simulink model "baselineisp_arch_v1"  (R2023b)
settings: Solver=VariableStepAuto  StartTime=0.0  StopTime=10.0  RelTol=1e-3
model workspace (MAT data in the model file):
  Input = Simulink.Bus
  Input.Alignment = -1
  Input.PreserveElementDimensions = 0
  Input.Elements_internal = Simulink.BusElement
  Input.Elements_internal.DimensionsMode = 'Fixed'
  Input.Elements_internal.SamplingMode = 'Sample based'
  Input.Elements_internal.SampleTime = -1
  Input.Elements_internal.Name = 'RAW'
  Input.Elements_internal.DataType_internal = 'ValueType: RAW'
  Input.Elements_internal.Complexity = 'real'
  Input.Elements_internal.Dimensions = 1
  Input.DataScope = 'Auto'
  RAW = Simulink.ValueType
  RAW.DataType = 'uint16'
settings Model: Creator=csl  LastModifiedBy=csl

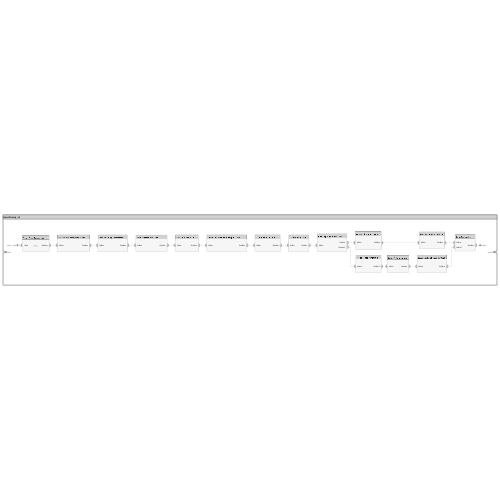
[thumbnail: Simulink's stored preview of the top-level diagram]
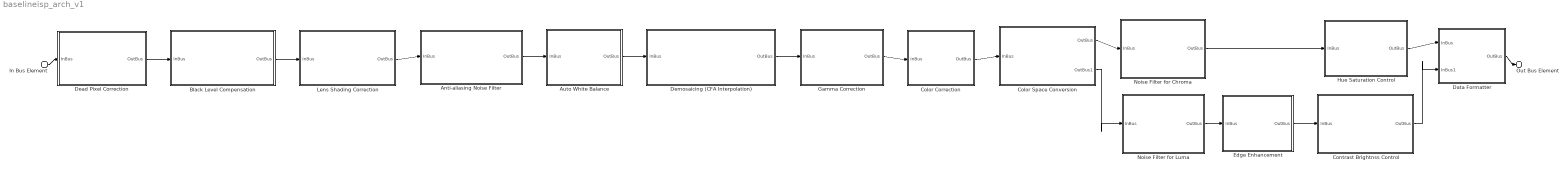
== system baselineisp_arch_v1 ==
  In Bus Element : Inport  PortName=InBus  Element=RAW
  Anti-aliasing Noise Filter : Subsystem
      settings: PortSchema="{\"entries\":[{\"content\":{\"headerSize\":26,\"margin\":15,\"minimumSpacing\":25,\"sides\":[{\"content\":{\"connectorIds\":[\"In1\"]},\"type\":\"ConnectorPlacement.EquallySpacedRectSide\",\"uuid\":\"2ef9bd17-36b9-46a7-9186-123a5b4f1bb0\"},{\"content\":{\"connectorIds\":[\"Out1\"],\"side\":\"RIGHT\"},\"type\":\"ConnectorPlacement.EquallySpacedRectSide\",\"uuid\":\"d5e57a0a-cb8d-4d21-83db-117ffcc7e54f\"},{\"content\":{\"side\":\"TOP\"},\"type\":\"ConnectorPlacement.EquallySpacedRectSide\",\"uuid\":\"a9269390-9b6c-4e98-a738-6052543cf38e\"}]},\"type\":\"ConnectorPlacement.EquallySpacedConnector\",\"uuid\":\"34a5eba8-ed92-482b-8745-835516add4be\"}],\"packageUris\":[\"http://schema.mathworks.com/mf0/Connector/R2020b\"],\"version\":\"1.0\"}"
  Auto White Balance : Subsystem
      settings: PortSchema="{\"entries\":[{\"content\":{\"headerSize\":26,\"margin\":15,\"minimumSpacing\":25,\"sides\":[{\"content\":{\"connectorIds\":[\"In1\"]},\"type\":\"ConnectorPlacement.EquallySpacedRectSide\",\"uuid\":\"2ef9bd17-36b9-46a7-9186-123a5b4f1bb0\"},{\"content\":{\"connectorIds\":[\"Out1\"],\"side\":\"RIGHT\"},\"type\":\"ConnectorPlacement.EquallySpacedRectSide\",\"uuid\":\"d5e57a0a-cb8d-4d21-83db-117ffcc7e54f\"},{\"content\":{\"side\":\"TOP\"},\"type\":\"ConnectorPlacement.EquallySpacedRectSide\",\"uuid\":\"a9269390-9b6c-4e98-a738-6052543cf38e\"},{\"content\":{\"side\":\"BOTTOM\"},\"type\":\"ConnectorPlacement.EquallySpacedRectSide\",\"uuid\":\"7c626892-77ff-47ce-8fd5-626703806efa\"}]},\"type\":\"ConnectorPlacement.EquallySpacedConnector\",\"uuid\":\"34a5eba8-ed92-482b-8745-835516add4be\"}],\"packageUris\":[\"http://schema.mathworks.com/mf0/Connector/R2020b\"],\"version\":\"1.0\"}"
  Black Level Compensation : Subsystem
      settings: PortSchema="{\"entries\":[{\"content\":{\"headerSize\":26,\"margin\":15,\"minimumSpacing\":25,\"sides\":[{\"content\":{\"connectorIds\":[\"In1\"]},\"type\":\"ConnectorPlacement.EquallySpacedRectSide\",\"uuid\":\"2ef9bd17-36b9-46a7-9186-123a5b4f1bb0\"},{\"content\":{\"connectorIds\":[\"Out1\"],\"side\":\"RIGHT\"},\"type\":\"ConnectorPlacement.EquallySpacedRectSide\",\"uuid\":\"d5e57a0a-cb8d-4d21-83db-117ffcc7e54f\"},{\"content\":{\"side\":\"TOP\"},\"type\":\"ConnectorPlacement.EquallySpacedRectSide\",\"uuid\":\"a9269390-9b6c-4e98-a738-6052543cf38e\"}]},\"type\":\"ConnectorPlacement.EquallySpacedConnector\",\"uuid\":\"34a5eba8-ed92-482b-8745-835516add4be\"}],\"packageUris\":[\"http://schema.mathworks.com/mf0/Connector/R2020b\"],\"version\":\"1.0\"}"
  Color Correction : Subsystem
      settings: PortSchema="{\"entries\":[{\"content\":{\"headerSize\":26,\"margin\":15,\"minimumSpacing\":25,\"sides\":[{\"content\":{\"connectorIds\":[\"In1\"]},\"type\":\"ConnectorPlacement.EquallySpacedRectSide\",\"uuid\":\"2ef9bd17-36b9-46a7-9186-123a5b4f1bb0\"},{\"content\":{\"connectorIds\":[\"Out1\"],\"side\":\"RIGHT\"},\"type\":\"ConnectorPlacement.EquallySpacedRectSide\",\"uuid\":\"d5e57a0a-cb8d-4d21-83db-117ffcc7e54f\"},{\"content\":{\"side\":\"TOP\"},\"type\":\"ConnectorPlacement.EquallySpacedRectSide\",\"uuid\":\"a9269390-9b6c-4e98-a738-6052543cf38e\"},{\"content\":{\"side\":\"BOTTOM\"},\"type\":\"ConnectorPlacement.EquallySpacedRectSide\",\"uuid\":\"3fcc8b46-bf35-454b-b542-ea93b895bca3\"}]},\"type\":\"ConnectorPlacement.EquallySpacedConnector\",\"uuid\":\"34a5eba8-ed92-482b-8745-835516add4be\"}],\"packageUris\":[\"http://schema.mathworks.com/mf0/Connector/R2020b\"],\"version\":\"1.0\"}"
  Color Space Conversion : Subsystem
      settings: PortSchema="{\"entries\":[{\"content\":{\"headerSize\":26,\"margin\":15,\"minimumSpacing\":25,\"sides\":[{\"content\":{\"connectorIds\":[\"In1\"]},\"type\":\"ConnectorPlacement.EquallySpacedRectSide\",\"uuid\":\"2ef9bd17-36b9-46a7-9186-123a5b4f1bb0\"},{\"content\":{\"connectorIds\":[\"Out1\",\"Out2\"],\"side\":\"RIGHT\"},\"type\":\"ConnectorPlacement.EquallySpacedRectSide\",\"uuid\":\"d5e57a0a-cb8d-4d21-83db-117ffcc7e54f\"},{\"content\":{\"side\":\"TOP\"},\"type\":\"ConnectorPlacement.EquallySpacedRectSide\",\"uuid\":\"a9269390-9b6c-4e98-a738-6052543cf38e\"}]},\"type\":\"ConnectorPlacement.EquallySpacedConnector\",\"uuid\":\"34a5eba8-ed92-482b-8745-835516add4be\"}],\"packageUris\":[\"http://schema.mathworks.com/mf0/Connector/R2020b\"],\"version\":\"1.0\"}"
  Contrast Brightnss Control : Subsystem
      settings: PortSchema="{\"entries\":[{\"content\":{\"headerSize\":26,\"margin\":15,\"minimumSpacing\":25,\"sides\":[{\"content\":{\"connectorIds\":[\"In1\"]},\"type\":\"ConnectorPlacement.EquallySpacedRectSide\",\"uuid\":\"2ef9bd17-36b9-46a7-9186-123a5b4f1bb0\"},{\"content\":{\"connectorIds\":[\"Out1\"],\"side\":\"RIGHT\"},\"type\":\"ConnectorPlacement.EquallySpacedRectSide\",\"uuid\":\"d5e57a0a-cb8d-4d21-83db-117ffcc7e54f\"},{\"content\":{\"side\":\"TOP\"},\"type\":\"ConnectorPlacement.EquallySpacedRectSide\",\"uuid\":\"a9269390-9b6c-4e98-a738-6052543cf38e\"}]},\"type\":\"ConnectorPlacement.EquallySpacedConnector\",\"uuid\":\"34a5eba8-ed92-482b-8745-835516add4be\"}],\"packageUris\":[\"http://schema.mathworks.com/mf0/Connector/R2020b\"],\"version\":\"1.0\"}"
  Data Formatter : Subsystem
      settings: PortSchema="{\"entries\":[{\"content\":{\"headerSize\":26,\"margin\":15,\"minimumSpacing\":25,\"sides\":[{\"content\":{\"connectorIds\":[\"In1\",\"In2\"]},\"type\":\"ConnectorPlacement.EquallySpacedRectSide\",\"uuid\":\"2ef9bd17-36b9-46a7-9186-123a5b4f1bb0\"},{\"content\":{\"connectorIds\":[\"Out1\"],\"side\":\"RIGHT\"},\"type\":\"ConnectorPlacement.EquallySpacedRectSide\",\"uuid\":\"d5e57a0a-cb8d-4d21-83db-117ffcc7e54f\"},{\"content\":{\"side\":\"TOP\"},\"type\":\"ConnectorPlacement.EquallySpacedRectSide\",\"uuid\":\"a9269390-9b6c-4e98-a738-6052543cf38e\"}]},\"type\":\"ConnectorPlacement.EquallySpacedConnector\",\"uuid\":\"34a5eba8-ed92-482b-8745-835516add4be\"}],\"packageUris\":[\"http://schema.mathworks.com/mf0/Connector/R2020b\"],\"version\":\"1.0\"}"
  Dead Pixel Correction : Subsystem
      settings: PortSchema="{\"entries\":[{\"content\":{\"headerSize\":26,\"margin\":15,\"minimumSpacing\":25,\"sides\":[{\"content\":{\"connectorIds\":[\"In1\"]},\"type\":\"ConnectorPlacement.EquallySpacedRectSide\",\"uuid\":\"2ef9bd17-36b9-46a7-9186-123a5b4f1bb0\"},{\"content\":{\"connectorIds\":[\"Out1\"],\"side\":\"RIGHT\"},\"type\":\"ConnectorPlacement.EquallySpacedRectSide\",\"uuid\":\"d5e57a0a-cb8d-4d21-83db-117ffcc7e54f\"},{\"content\":{\"side\":\"TOP\"},\"type\":\"ConnectorPlacement.EquallySpacedRectSide\",\"uuid\":\"a9269390-9b6c-4e98-a738-6052543cf38e\"}]},\"type\":\"ConnectorPlacement.EquallySpacedConnector\",\"uuid\":\"34a5eba8-ed92-482b-8745-835516add4be\"}],\"packageUris\":[\"http://schema.mathworks.com/mf0/Connector/R2020b\"],\"version\":\"1.0\"}"
  Demosaicing (CFA Interpolation) : Subsystem
      settings: PortSchema="{\"entries\":[{\"content\":{\"headerSize\":26,\"margin\":15,\"minimumSpacing\":25,\"sides\":[{\"content\":{\"connectorIds\":[\"In1\"]},\"type\":\"ConnectorPlacement.EquallySpacedRectSide\",\"uuid\":\"2ef9bd17-36b9-46a7-9186-123a5b4f1bb0\"},{\"content\":{\"connectorIds\":[\"Out1\"],\"side\":\"RIGHT\"},\"type\":\"ConnectorPlacement.EquallySpacedRectSide\",\"uuid\":\"d5e57a0a-cb8d-4d21-83db-117ffcc7e54f\"},{\"content\":{\"side\":\"TOP\"},\"type\":\"ConnectorPlacement.EquallySpacedRectSide\",\"uuid\":\"a9269390-9b6c-4e98-a738-6052543cf38e\"}]},\"type\":\"ConnectorPlacement.EquallySpacedConnector\",\"uuid\":\"34a5eba8-ed92-482b-8745-835516add4be\"}],\"packageUris\":[\"http://schema.mathworks.com/mf0/Connector/R2020b\"],\"version\":\"1.0\"}"
  Edge Enhancement : Subsystem
      settings: PortSchema="{\"entries\":[{\"content\":{\"headerSize\":26,\"margin\":15,\"minimumSpacing\":25,\"sides\":[{\"content\":{\"connectorIds\":[\"In1\"]},\"type\":\"ConnectorPlacement.EquallySpacedRectSide\",\"uuid\":\"2ef9bd17-36b9-46a7-9186-123a5b4f1bb0\"},{\"content\":{\"connectorIds\":[\"Out1\"],\"side\":\"RIGHT\"},\"type\":\"ConnectorPlacement.EquallySpacedRectSide\",\"uuid\":\"d5e57a0a-cb8d-4d21-83db-117ffcc7e54f\"},{\"content\":{\"side\":\"TOP\"},\"type\":\"ConnectorPlacement.EquallySpacedRectSide\",\"uuid\":\"a9269390-9b6c-4e98-a738-6052543cf38e\"}]},\"type\":\"ConnectorPlacement.EquallySpacedConnector\",\"uuid\":\"34a5eba8-ed92-482b-8745-835516add4be\"}],\"packageUris\":[\"http://schema.mathworks.com/mf0/Connector/R2020b\"],\"version\":\"1.0\"}"
  Gamma Correction : Subsystem
      settings: PortSchema="{\"entries\":[{\"content\":{\"headerSize\":26,\"margin\":15,\"minimumSpacing\":25,\"sides\":[{\"content\":{\"connectorIds\":[\"In1\"]},\"type\":\"ConnectorPlacement.EquallySpacedRectSide\",\"uuid\":\"2ef9bd17-36b9-46a7-9186-123a5b4f1bb0\"},{\"content\":{\"connectorIds\":[\"Out1\"],\"side\":\"RIGHT\"},\"type\":\"ConnectorPlacement.EquallySpacedRectSide\",\"uuid\":\"d5e57a0a-cb8d-4d21-83db-117ffcc7e54f\"},{\"content\":{\"side\":\"TOP\"},\"type\":\"ConnectorPlacement.EquallySpacedRectSide\",\"uuid\":\"a9269390-9b6c-4e98-a738-6052543cf38e\"},{\"content\":{\"side\":\"BOTTOM\"},\"type\":\"ConnectorPlacement.EquallySpacedRectSide\",\"uuid\":\"141ec45e-843e-4f7e-bcc3-8daa426655ca\"}]},\"type\":\"ConnectorPlacement.EquallySpacedConnector\",\"uuid\":\"34a5eba8-ed92-482b-8745-835516add4be\"}],\"packageUris\":[\"http://schema.mathworks.com/mf0/Connector/R2020b\"],\"version\":\"1.0\"}"
  Hue Saturation Control : Subsystem
      settings: PortSchema="{\"entries\":[{\"content\":{\"headerSize\":26,\"margin\":15,\"minimumSpacing\":25,\"sides\":[{\"content\":{\"connectorIds\":[\"In1\"]},\"type\":\"ConnectorPlacement.EquallySpacedRectSide\",\"uuid\":\"2ef9bd17-36b9-46a7-9186-123a5b4f1bb0\"},{\"content\":{\"connectorIds\":[\"Out1\"],\"side\":\"RIGHT\"},\"type\":\"ConnectorPlacement.EquallySpacedRectSide\",\"uuid\":\"d5e57a0a-cb8d-4d21-83db-117ffcc7e54f\"},{\"content\":{\"side\":\"TOP\"},\"type\":\"ConnectorPlacement.EquallySpacedRectSide\",\"uuid\":\"a9269390-9b6c-4e98-a738-6052543cf38e\"}]},\"type\":\"ConnectorPlacement.EquallySpacedConnector\",\"uuid\":\"34a5eba8-ed92-482b-8745-835516add4be\"}],\"packageUris\":[\"http://schema.mathworks.com/mf0/Connector/R2020b\"],\"version\":\"1.0\"}"
  Lens Shading Correction : Subsystem
      settings: PortSchema="{\"entries\":[{\"content\":{\"headerSize\":26,\"margin\":15,\"minimumSpacing\":25,\"sides\":[{\"content\":{\"connectorIds\":[\"In1\"]},\"type\":\"ConnectorPlacement.EquallySpacedRectSide\",\"uuid\":\"2ef9bd17-36b9-46a7-9186-123a5b4f1bb0\"},{\"content\":{\"connectorIds\":[\"Out1\"],\"side\":\"RIGHT\"},\"type\":\"ConnectorPlacement.EquallySpacedRectSide\",\"uuid\":\"d5e57a0a-cb8d-4d21-83db-117ffcc7e54f\"},{\"content\":{\"side\":\"TOP\"},\"type\":\"ConnectorPlacement.EquallySpacedRectSide\",\"uuid\":\"a9269390-9b6c-4e98-a738-6052543cf38e\"}]},\"type\":\"ConnectorPlacement.EquallySpacedConnector\",\"uuid\":\"34a5eba8-ed92-482b-8745-835516add4be\"}],\"packageUris\":[\"http://schema.mathworks.com/mf0/Connector/R2020b\"],\"version\":\"1.0\"}"
  Noise Filter for Chroma : Subsystem
      settings: PortSchema="{\"entries\":[{\"content\":{\"headerSize\":26,\"margin\":15,\"minimumSpacing\":25,\"sides\":[{\"content\":{\"connectorIds\":[\"In1\"]},\"type\":\"ConnectorPlacement.EquallySpacedRectSide\",\"uuid\":\"2ef9bd17-36b9-46a7-9186-123a5b4f1bb0\"},{\"content\":{\"connectorIds\":[\"Out1\"],\"side\":\"RIGHT\"},\"type\":\"ConnectorPlacement.EquallySpacedRectSide\",\"uuid\":\"d5e57a0a-cb8d-4d21-83db-117ffcc7e54f\"},{\"content\":{\"side\":\"TOP\"},\"type\":\"ConnectorPlacement.EquallySpacedRectSide\",\"uuid\":\"a9269390-9b6c-4e98-a738-6052543cf38e\"}]},\"type\":\"ConnectorPlacement.EquallySpacedConnector\",\"uuid\":\"34a5eba8-ed92-482b-8745-835516add4be\"}],\"packageUris\":[\"http://schema.mathworks.com/mf0/Connector/R2020b\"],\"version\":\"1.0\"}"
  Noise Filter for Luma : Subsystem
      settings: PortSchema="{\"entries\":[{\"content\":{\"headerSize\":26,\"margin\":15,\"minimumSpacing\":25,\"sides\":[{\"content\":{\"connectorIds\":[\"In1\"]},\"type\":\"ConnectorPlacement.EquallySpacedRectSide\",\"uuid\":\"2ef9bd17-36b9-46a7-9186-123a5b4f1bb0\"},{\"content\":{\"connectorIds\":[\"Out1\"],\"side\":\"RIGHT\"},\"type\":\"ConnectorPlacement.EquallySpacedRectSide\",\"uuid\":\"d5e57a0a-cb8d-4d21-83db-117ffcc7e54f\"},{\"content\":{\"side\":\"TOP\"},\"type\":\"ConnectorPlacement.EquallySpacedRectSide\",\"uuid\":\"a9269390-9b6c-4e98-a738-6052543cf38e\"}]},\"type\":\"ConnectorPlacement.EquallySpacedConnector\",\"uuid\":\"34a5eba8-ed92-482b-8745-835516add4be\"}],\"packageUris\":[\"http://schema.mathworks.com/mf0/Connector/R2020b\"],\"version\":\"1.0\"}"
  Out Bus Element : Outport  PortName=OutBus
  wires:
  Data Formatter/1(OutBus) -> Out Bus Element/1
  Contrast Brightnss Control/1(OutBus) -> Data Formatter/2(InBus1)
  Hue Saturation Control/1(OutBus) -> Data Formatter/1(InBus)
  Edge Enhancement/1(OutBus) -> Contrast Brightnss Control/1(InBus)
  In Bus Element/1 -> Dead Pixel Correction/1(InBus)
  Color Space Conversion/1(OutBus) -> Noise Filter for Chroma/1(InBus)
  Dead Pixel Correction/1(OutBus) -> Black Level Compensation/1(InBus)
  Black Level Compensation/1(OutBus) -> Lens Shading Correction/1(InBus)
  Lens Shading Correction/1(OutBus) -> Anti-aliasing Noise Filter/1(InBus)
  Anti-aliasing Noise Filter/1(OutBus) -> Auto White Balance/1(InBus)
  Auto White Balance/1(OutBus) -> Demosaicing (CFA Interpolation)/1(InBus)
  Demosaicing (CFA Interpolation)/1(OutBus) -> Gamma Correction/1(InBus)
  Gamma Correction/1(OutBus) -> Color Correction/1(InBus)
  Noise Filter for Luma/1(OutBus) -> Edge Enhancement/1(InBus)
  Color Correction/1(OutBus) -> Color Space Conversion/1(InBus)
  Noise Filter for Chroma/1(OutBus) -> Hue Saturation Control/1(InBus)
  Color Space Conversion/2(OutBus1) -> Noise Filter for Luma/1(InBus)

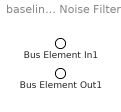
== system baselineisp_arch_v1/Anti-aliasing Noise Filter ==
  Bus Element In1 : Inport  PortName=InBus
  Bus Element Out1 : Outport  PortName=OutBus

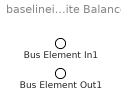
== system baselineisp_arch_v1/Auto White Balance ==
  Bus Element In1 : Inport  PortName=InBus
  Bus Element Out1 : Outport  PortName=OutBus

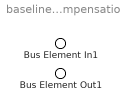
== system baselineisp_arch_v1/Black Level Compensation ==
  Bus Element In1 : Inport  PortName=InBus
  Bus Element Out1 : Outport  PortName=OutBus

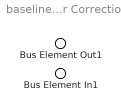
== system baselineisp_arch_v1/Color Correction ==
  Bus Element In1 : Inport  PortName=InBus
  Bus Element Out1 : Outport  PortName=OutBus

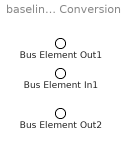
== system baselineisp_arch_v1/Color Space Conversion ==
  Bus Element In1 : Inport  PortName=InBus
  Bus Element Out1 : Outport  PortName=OutBus
  Bus Element Out2 : Outport  Port=2  PortName=OutBus1

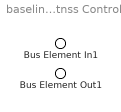
== system baselineisp_arch_v1/Contrast Brightnss Control ==
  Bus Element In1 : Inport  PortName=InBus
  Bus Element Out1 : Outport  PortName=OutBus

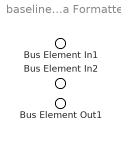
== system baselineisp_arch_v1/Data Formatter ==
  Bus Element In1 : Inport  PortName=InBus
  Bus Element In2 : Inport  Port=2  PortName=InBus1
  Bus Element Out1 : Outport  PortName=OutBus

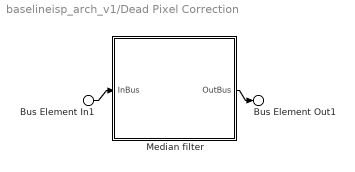
== system baselineisp_arch_v1/Dead Pixel Correction ==
  Bus Element In1 : Inport  PortName=InBus
  Median filter : Subsystem
      settings: PortSchema="{\"entries\":[{\"content\":{\"headerSize\":26,\"margin\":15,\"minimumSpacing\":25,\"sides\":[{\"content\":{\"connectorIds\":[\"In1\"]},\"type\":\"ConnectorPlacement.EquallySpacedRectSide\",\"uuid\":\"076aee67-dc06-437d-bc64-528b33023a13\"},{\"content\":{\"connectorIds\":[\"Out1\"],\"side\":\"RIGHT\"},\"type\":\"ConnectorPlacement.EquallySpacedRectSide\",\"uuid\":\"a939dd39-aae9-418d-93c0-dbd8279e83bb\"},{\"content\":{\"side\":\"TOP\"},\"type\":\"ConnectorPlacement.EquallySpacedRectSide\",\"uuid\":\"0722a1d4-3145-4f42-9c90-bf1b84f9c478\"}]},\"type\":\"ConnectorPlacement.EquallySpacedConnector\",\"uuid\":\"3d792aeb-9d60-4cc3-971e-83e92acc61e6\"}],\"packageUris\":[\"http://schema.mathworks.com/mf0/Connector/R2020b\"],\"version\":\"1.0\"}"
  Bus Element Out1 : Outport  PortName=OutBus
  wires:
  Bus Element In1/1 -> Median filter/1(InBus)
  Median filter/1(OutBus) -> Bus Element Out1/1

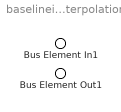
== system baselineisp_arch_v1/Demosaicing (CFA Interpolation) ==
  Bus Element In1 : Inport  PortName=InBus
  Bus Element Out1 : Outport  PortName=OutBus

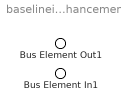
== system baselineisp_arch_v1/Edge Enhancement ==
  Bus Element In1 : Inport  PortName=InBus
  Bus Element Out1 : Outport  PortName=OutBus

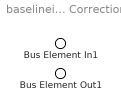
== system baselineisp_arch_v1/Gamma Correction ==
  Bus Element In1 : Inport  PortName=InBus
  Bus Element Out1 : Outport  PortName=OutBus

== system baselineisp_arch_v1/Hue Saturation Control ==
  Bus Element In1 : Inport  PortName=InBus
  Bus Element Out1 : Outport  PortName=OutBus

== system baselineisp_arch_v1/Lens Shading Correction ==
  Bus Element In1 : Inport  PortName=InBus
  Bus Element Out1 : Outport  PortName=OutBus

== system baselineisp_arch_v1/Noise Filter for Chroma ==
  Bus Element In1 : Inport  PortName=InBus
  Bus Element Out1 : Outport  PortName=OutBus

== system baselineisp_arch_v1/Noise Filter for Luma ==
  Bus Element In1 : Inport  PortName=InBus
  Bus Element Out1 : Outport  PortName=OutBus

== system baselineisp_arch_v1/Dead Pixel Correction/Median filter ==
  Bus Element In1 : Inport  PortName=InBus
  Bus Element Out1 : Outport  PortName=OutBus
